simulink model "path_following_baseline"  (R2026a)
settings: Solver=ode4  StopTime=15  FixedStep=1e-3
PreLoadFcn:
  | addpath(fullfile(fileparts(which('path_following_baseline')), 'src')); init_model_workspace;
values from neighbouring files (symbols this model uses):
  xy_monitor_on = 0    [my_design_template.m]    (also in run_baseline.m)
undefined symbols (not defined in the file or in its folder): delta_max, K, pth_vec, Ts_mon, veh, Vx
libraries: autolibshared x1
Description:
  | Baseline project: vehicle path-following control of an S-shaped lane change with full-state feedback (Vehicle Body 3DOF Single Track plant).
settings Model: Creator=lemon  LastModifiedBy=lemon

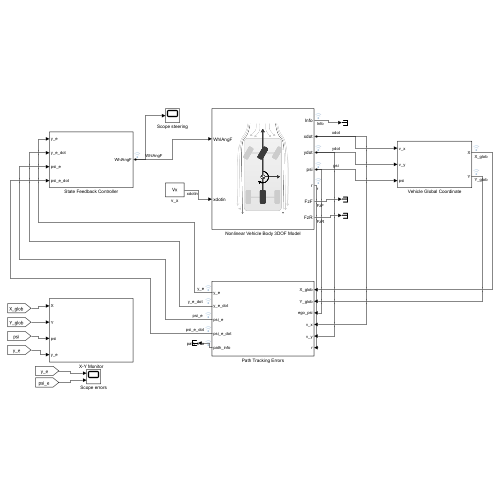
[thumbnail: Simulink's stored preview of the top-level diagram]
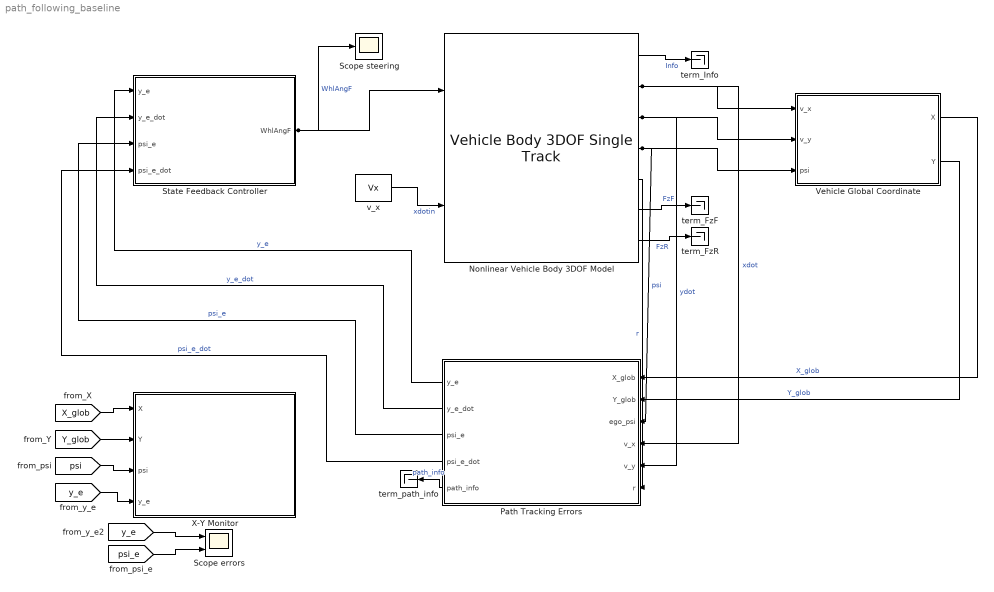
== system path_following_baseline ==
  Nonlinear Vehicle Body 3DOF Model : autolibshared/Vehicle Body 3DOF Single Track  trackMode=Single (bicycle)  inputMode=External longitudinal velocity  frontSteerMode=on  rearSteerMode=off  extFMode=off  htchFMode=off  extMMode=off  htchMMode=off  windMode=off  extTamb=off  muMode=off  extGndPlnElev=off  extGndPlnRoll=off  extGndPlnPitch=off  extGndPlnDCM=off  extXo=off  extxdoto=off  extYo=off  extydoto=off  extpsio=off  extro=off  aMode=2  NF=2  NR=2  m=veh.m  a=veh.lf  b=veh.lr  h=0.35  dh=1  hh=0.2  X_o=0  xdot_o=0  d=0  hl=0  w=[1.4,1.4]  CalphaMode=Constant  sigmaMode=on  sigma_f=.1  sigma_r=.1  Cy_f=blk.Cy_f  Cy_r=blk.Cy_r  Cy_f_data="[1.396121365092108e+04\t4.232462640127975e+04\t6.754894575573687e+04\t8.835784428391886e+04\t1.043551700699839e+05\t1.158335754468729e+05\t1.234691551560788e+05\t1.280575366661118e+05\t1.298126639907242e+05\t1.298126639907242e+05]"  alpha_f_brk=[-0.785, -0.628, -0.471, -0.314, -0.157, 0.000, 0.157, 0.314, 0.471, 0.628, 0.785]  Fz_f_brk="[500\t1.555555555555556e+03\t2.611111111111111e+03\t3.666666666666667e+03\t4.722222222222223e+03\t5.777777777777777e+03\t6.833333333333333e+03\t7.888888888888889e+03\t8.944444444444445e+03\t10000]"  Cy_r_data="[1.396121365092108e+04\t4.232462640127975e+04\t6.754894575573687e+04\t8.835784428391886e+04\t1.043551700699839e+05\t1.158335754468729e+05\t1.234691551560788e+05\t1.280575366661118e+05\t1.298126639907242e+05\t1.298126639907242e+05]"  alpha_r_brk=[-0.785, -0.628, -0.471, -0.314, -0.157, 0.000, 0.157, 0.314, 0.471, 0.628, 0.785]  Fz_r_brk="[500\t1.555555555555556e+03\t2.611111111111111e+03\t3.666666666666667e+03\t4.722222222222223e+03\t5.777777777777777e+03\t6.833333333333333e+03\t7.888888888888889e+03\t8.944444444444445e+03\t10000]"  Fznom=blk.Fznom  Y_o=0  ydot_o=0  Izz=veh.Izz  psi_o=0  r_o=0  Af=2  Cd=blk.Cd  Cl=blk.Cl  Cpm=blk.Cpm  beta_w=[0 0.01:0.01:0.3]  Cs=[0 0.01:0.01:0.3]  Cym=[0 1e-6:0.01:0.3]  Pabs=101325  Tair=273  g=veh.g  mu=1  GndPlnRoll=0  GndPlnPitch=0  GndPlnElev=0  xdot_tol=.01  Fxtire_sat=7e4  Fytire_sat=7e4  longOff=0  latOff=0  vertOff=0.35  wrapAng=off
  Path Tracking Errors : Subsystem
  Scope errors : Scope  NumInputPorts=2
  Scope steering : Scope
  State Feedback Controller : Subsystem
  Vehicle Global Coordinate : Subsystem
  X-Y Monitor : Subsystem
  term_FzF : Terminator
  term_FzR : Terminator
  term_Info : Terminator
  term_path_info : Terminator
  v_x : Constant  Value=Vx
  wires:
  State Feedback Controller/1(WhlAngF) -> Nonlinear Vehicle Body 3DOF Model/1, Scope steering/1  "WhlAngF"
  v_x/1 -> Nonlinear Vehicle Body 3DOF Model/2  "xdotin"
  Nonlinear Vehicle Body 3DOF Model/1 -> term_Info/1  "Info"
  Nonlinear Vehicle Body 3DOF Model/2 -> Vehicle Global Coordinate/1(v_x), Path Tracking Errors/4(v_x)  "xdot"
  Nonlinear Vehicle Body 3DOF Model/3 -> Vehicle Global Coordinate/2(v_y), Path Tracking Errors/5(v_y)  "ydot"
  Nonlinear Vehicle Body 3DOF Model/4 -> Vehicle Global Coordinate/3(psi), Path Tracking Errors/3(ego_psi)  "psi"
  Nonlinear Vehicle Body 3DOF Model/5 -> Path Tracking Errors/6(r)  "r"
  Nonlinear Vehicle Body 3DOF Model/6 -> term_FzF/1  "FzF"
  Nonlinear Vehicle Body 3DOF Model/7 -> term_FzR/1  "FzR"
  Vehicle Global Coordinate/1(X) -> Path Tracking Errors/1(X_glob)  "X_glob"
  Vehicle Global Coordinate/2(Y) -> Path Tracking Errors/2(Y_glob)  "Y_glob"
  Path Tracking Errors/1(y_e) -> State Feedback Controller/1(y_e)  "y_e"
  Path Tracking Errors/2(y_e_dot) -> State Feedback Controller/2(y_e_dot)  "y_e_dot"
  Path Tracking Errors/3(psi_e) -> State Feedback Controller/3(psi_e)  "psi_e"
  Path Tracking Errors/4(psi_e_dot) -> State Feedback Controller/4(psi_e_dot)  "psi_e_dot"
  Path Tracking Errors/5(path_info) -> term_path_info/1  "path_info"
  [X_glob] -> X-Y Monitor/1(X)
  [Y_glob] -> X-Y Monitor/2(Y)
  [psi] -> X-Y Monitor/3(psi)
  [y_e] -> X-Y Monitor/4(y_e)
  [y_e] -> Scope errors/1
  [psi_e] -> Scope errors/2

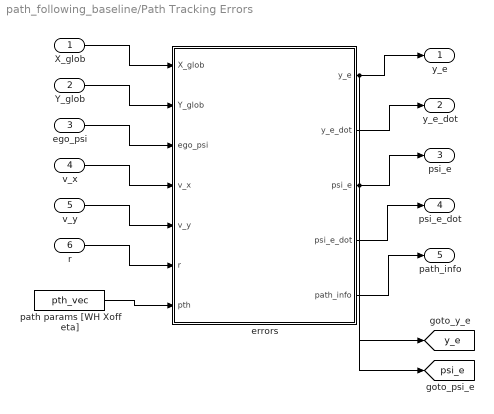
== system path_following_baseline/Path Tracking Errors ==
  X_glob : Inport
  Y_glob : Inport  Port=2
  ego_psi : Inport  Port=3
  v_x : Inport  Port=4
  v_y : Inport  Port=5
  r : Inport  Port=6
  errors : MATLAB Function  TreatAsAtomicUnit=on
  path params [WH Xoff eta] : Constant  Value=pth_vec
  y_e : Outport
  y_e_dot : Outport  Port=2
  psi_e : Outport  Port=3
  psi_e_dot : Outport  Port=4
  path_info : Outport  Port=5
  tag scope: psi_e=global, y_e=global
  wires:
  X_glob/1 -> errors/1(X_glob)
  Y_glob/1 -> errors/2(Y_glob)
  ego_psi/1 -> errors/3(ego_psi)
  v_x/1 -> errors/4(v_x)
  v_y/1 -> errors/5(v_y)
  r/1 -> errors/6(r)
  path params [WH Xoff eta]/1 -> errors/7(pth)
  errors/1(y_e) -> y_e/1, [y_e]
  errors/2(y_e_dot) -> y_e_dot/1
  errors/3(psi_e) -> psi_e/1, [psi_e]
  errors/4(psi_e_dot) -> psi_e_dot/1
  errors/5(path_info) -> path_info/1

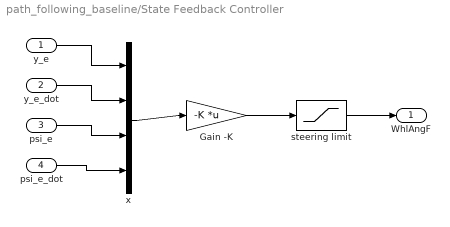
== system path_following_baseline/State Feedback Controller ==
  y_e : Inport
  y_e_dot : Inport  Port=2
  psi_e : Inport  Port=3
  psi_e_dot : Inport  Port=4
  Gain -K : Gain  Gain=-K  Multiplication=Matrix(K*u)
  steering limit : Saturate  UpperLimit=delta_max  LowerLimit=-delta_max
  x : Mux
  WhlAngF : Outport
  wires:
  y_e/1 -> x/1
  y_e_dot/1 -> x/2
  psi_e/1 -> x/3
  psi_e_dot/1 -> x/4
  x/1 -> Gain -K/1
  Gain -K/1 -> steering limit/1
  steering limit/1 -> WhlAngF/1

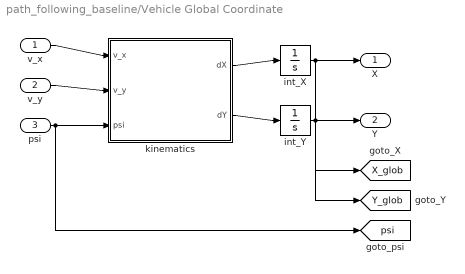
== system path_following_baseline/Vehicle Global Coordinate ==
  v_x : Inport
  v_y : Inport  Port=2
  psi : Inport  Port=3
  int_X : Integrator
  int_Y : Integrator
  kinematics : MATLAB Function  TreatAsAtomicUnit=on
  X : Outport
  Y : Outport  Port=2
  tag scope: X_glob=global, Y_glob=global, psi=global
  wires:
  v_x/1 -> kinematics/1(v_x)
  v_y/1 -> kinematics/2(v_y)
  psi/1 -> kinematics/3(psi), [psi]
  kinematics/1(dX) -> int_X/1
  kinematics/2(dY) -> int_Y/1
  int_X/1 -> X/1, [X_glob]
  int_Y/1 -> Y/1, [Y_glob]

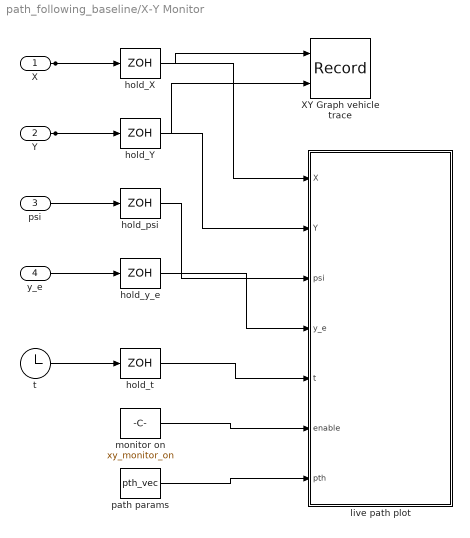
== system path_following_baseline/X-Y Monitor ==
  X : Inport
  Y : Inport  Port=2
  psi : Inport  Port=3
  y_e : Inport  Port=4
  XY Graph vehicle trace : Record  NumPorts=2.0  FileSettingsInternal="{\"entries\":[{\"content\":{\"excelSettings\":{\"content\":{},\"type\":\"Streamout.ExcelSettings\"},\"parquetSettings\":{\"content\":{},\"type\":\"Streamout.ParquetSettings\"}},\"type\":\"Streamout.FileSettingStorage\",\"uuid\":\"\"}],\"packageUris\":[\"http:\\/\\/schema.mathworks.com\\/mf0\\/streamout_blocks\\/R2020a\"],\"version\":\"1.0\"}"  FrameSettings=[0, 0]  Layout=[1 1]  SignalsInternal="{\"entries\":[{\"content\":{\"signals\":[{\"content\":{\"blockPath\":[],\"dimensions\":[1],\"domain\":\"\",\"lineColor\":\"#a2142f\",\"plots\":[ 1 ],\"port\":1,\"signalID\":1,\"signalName\":\"XY Graph:1\"},\"type\":\"RecordBlkView.Signal\",\"uuid\":\"\"},{\"content\":{\"blockPath\":[],\"dimensions\":[1],\"domain\":\"\",\"lineColor\":\"#139fff\",\"plots\":[ 1 ],\"port\":2,\"signalID\":2,\"signalName\":\"XY Graph:2\"},\"type\":\"RecordBlkView.Signal\",\"uuid\":\"\"}]},\"type\":\"RecordBlkView.InputSignals\",\"uuid\":\"\"}],\"packageUris\":[\"http:\\/\\/schema.mathworks.com\\/mf0\\/streamout_blocks\\/R2020a\"],\"version\":\"1.0\"}"  VisualizationBindings="{\"xyplotplugin\":{\"info\":[{\"series\":[{\"bindingParametersList\":[{\"parameter\":\"X-Axis\",\"signalID\":1,\"signalName\":\"XY Graph:1\"},{\"parameter\":\"Y-Axis\",\"signalID\":2,\"signalName\":\"XY Graph:2\"}],\"seriesID\":0}],\"subplotID\":1}]}}"  CompatibilityTag=XY
  hold_X : ZeroOrderHold  SampleTime=Ts_mon
  hold_Y : ZeroOrderHold  SampleTime=Ts_mon
  hold_psi : ZeroOrderHold  SampleTime=Ts_mon
  hold_t : ZeroOrderHold  SampleTime=Ts_mon
  hold_y_e : ZeroOrderHold  SampleTime=Ts_mon
  live path plot : MATLAB Function  TreatAsAtomicUnit=on
  monitor on : Constant  Value=xy_monitor_on
  path params : Constant  Value=pth_vec
  t : Clock
  wires:
  X/1 -> XY Graph vehicle trace/1, hold_X/1
  Y/1 -> XY Graph vehicle trace/2, hold_Y/1
  psi/1 -> hold_psi/1
  y_e/1 -> hold_y_e/1
  t/1 -> hold_t/1
  hold_X/1 -> live path plot/1(X)
  hold_Y/1 -> live path plot/2(Y)
  hold_psi/1 -> live path plot/3(psi)
  hold_y_e/1 -> live path plot/4(y_e)
  hold_t/1 -> live path plot/5(t)
  monitor on/1 -> live path plot/6(enable)
  path params/1 -> live path plot/7(pth)

== matlab function path_following_baseline/Path Tracking Errors/errors ==
  data: X_glob input; y_e output; Y_glob input; ego_psi input; v_x input; v_y input; r input; pth input; y_e_dot output; psi_e output; psi_e_dot output; path_info output
function [y_e, y_e_dot, psi_e, psi_e_dot, path_info] = errors(X_glob, Y_glob, ego_psi, v_x, v_y, r, pth)
%#codegen
% Lateral offset and heading error of the CG w.r.t. the S-shaped path
%   Y = WH*tanh((X - Xoff)/eta) + WH,   pth = [WH, Xoff, eta]
% path_info = [Xp, Yp, psi_p, kappa, psi_dot_des]  (see src/path_tracking_errors.m)
[y_e, y_e_dot, psi_e, psi_e_dot, path_info] = path_tracking_errors(X_glob, Y_glob, ego_psi, v_x, v_y, r, pth);

== matlab function path_following_baseline/Vehicle Global Coordinate/kinematics ==
  data: v_x input; dX output; v_y input; psi input; dY output
function [dX, dY] = kinematics(v_x, v_y, psi)
%#codegen
% Body-frame velocity -> inertial-frame velocity of the CG
% (see src/global_coordinate.m)
[dX, dY] = global_coordinate(v_x, v_y, psi);

== matlab function path_following_baseline/X-Y Monitor/live path plot ==
  data: X input; Y input; psi input; y_e input; t input; enable input; pth input
function live_path_plot(X, Y, psi, y_e, t, enable, pth)
%#codegen
% Animated X-Y monitor figure: reference path + vehicle CG trace + ego
% vehicle triangle (nose along the yaw angle psi).  Implemented in
% src/xy_monitor_update.m (called extrinsically, i.e. in MATLAB, every
% Ts_mon seconds).  Disabled when xy_monitor_on = 0.
coder.extrinsic('xy_monitor_update');
if enable > 0
    xy_monitor_update(t, X, Y, psi, y_e, pth);
end
